simulink model "simulation"  (R2016b)
settings: Solver=FixedStepAuto  StartTime=0.0  StopTime=15  FixedStep=0.05  RelTol=1e-3
values from neighbouring files (symbols this model uses):
  AccReqTable = [ ... (first row only)    [paras_table.m]
  CC_Delta_V_Pos = [0    0.5   1   2   5   10   20   30]    [paras_table.m]
  CC_P_Arr_Pos = [0.6  0.6  0.5 0.4 0.2  0.15 0.1 0.08]    [paras_table.m]
  Delta_Acc = [ 0   0.5  0.8  1.2  1.6 2.0 3.0 5.0]    [paras_table.m]
  DeltaSArr = [-40 -35 -30 -25 -20 -18 -16 -14 -12 -10 -8 -6 -4 -2 0 2 4 6 8 10 12 14 16 18 20 25 30 35 40 45 50 60 70 80 90]    [paras_table.m]
  DeltaVArr = [-30 -28 -26 -24 -22 -20 -18 -16 -14 -12 -10  -9  -8  -7  -6  -5 -4 -3 -2 -1 0 1 2 3 4  5  6  7  8 9  10 12 14 16 18 20 22 24 26 28 30]    [paras_table.m]
  Ego_Acc_arr = [2    2     2   1.5    1]    [paras_table.m]
  Ego_dece_arr = [-5  -5     -4   -3.5 -2.5]    [paras_table.m]
  Ego_V_arr = [0    5     10   20    30]    [paras_table.m]
  Neg_Jerk = [-4   -4  -2.5 -2  -1]    [paras_table.m]
  Pos_Jerk = [0.5  0.8  1.2  1.8  2.0 2.5 3.0 3.0]    [paras_table.m]
  TTC_Arr = [0    10   20  40 100]    [paras_table.m]
settings Model: Creator=Administrator  LastModifiedBy=Administrator

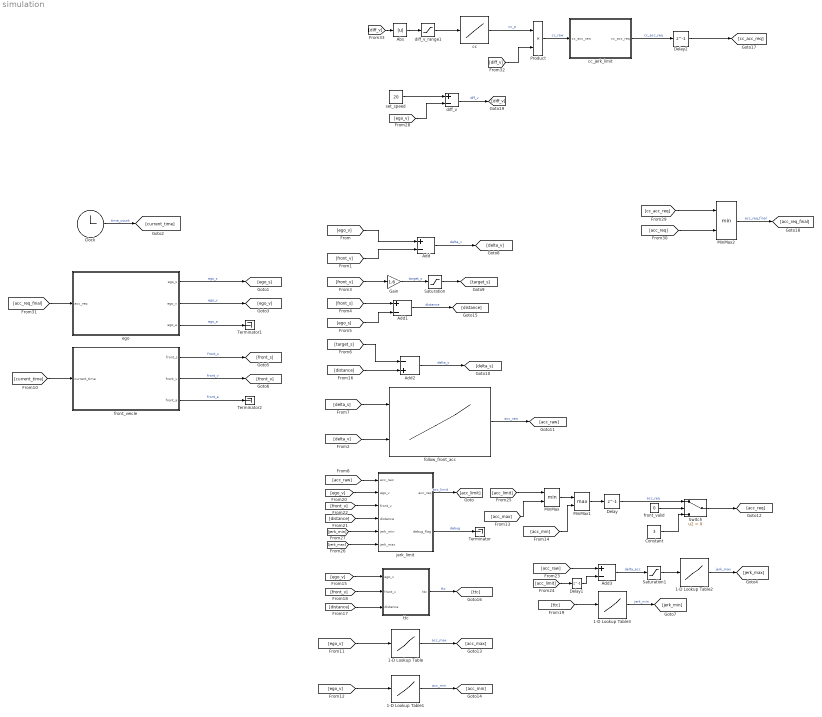
== system simulation ==
  1-D Lookup Table : Lookup_n-D  NumberOfTableDimensions=1  BreakpointsForDimension1=Ego_V_arr  Table=Ego_Acc_arr  InternalRulePriority=Speed  RndMeth=Simplest  InputSameDT=on
  1-D Lookup Table1 : Lookup_n-D  NumberOfTableDimensions=1  BreakpointsForDimension1=Ego_V_arr  Table=Ego_dece_arr  InternalRulePriority=Speed  RndMeth=Simplest  InputSameDT=on
  1-D Lookup Table2 : Lookup_n-D  NumberOfTableDimensions=1  BreakpointsForDimension1=Delta_Acc  Table=Pos_Jerk  InternalRulePriority=Speed  RndMeth=Simplest  InputSameDT=on
  1-D Lookup Table3 : Lookup_n-D  NumberOfTableDimensions=1  BreakpointsForDimension1=TTC_Arr  Table=Neg_Jerk  InternalRulePriority=Speed  RndMeth=Simplest  InputSameDT=on
  Abs : Abs
  Add : Sum  Inputs=+-
  Add1 : Sum  Inputs=+-
  Add2 : Sum  Inputs=-+
  Add3 : Sum  Inputs=+-
  Clock : Clock
  Constant : Constant  Value=3
  Delay : Delay  DelayLength=1  InitialCondition=0
  Delay1 : Delay  DelayLength=1  InitialCondition=0
  Delay2 : Delay  DelayLength=1  InitialCondition=0
  Gain : Gain  Gain=1.6
  MinMax : MinMax  Inputs=2
  MinMax1 : MinMax  Function=max  Inputs=2
  MinMax2 : MinMax  Inputs=2
  Product : Product
  Saturation : Saturate  UpperLimit=150  LowerLimit=3
  Saturation1 : Saturate  UpperLimit=5  LowerLimit=0
  Switch : Switch  Criteria=u2 > Threshold
  Terminator : Terminator
  Terminator1 : Terminator
  Terminator2 : Terminator
  cc : Lookup_n-D  NumberOfTableDimensions=1  BreakpointsForDimension1=CC_Delta_V_Pos  IndexSearchMethod=Linear search  Table=CC_P_Arr_Pos  InternalRulePriority=Speed  RndMeth=Simplest  InputSameDT=on
  cc_jerk_limit : MATLAB Function  TreatAsAtomicUnit=on
  diff_v : Sum  Inputs=+-
  diff_v_range1 : Saturate  UpperLimit=30  LowerLimit=0
  ego : MATLAB Function  TreatAsAtomicUnit=on
  "follow_front_acc " : Lookup_n-D  BreakpointsForDimension1=DeltaSArr  BreakpointsForDimension2=DeltaVArr  Table=AccReqTable  InternalRulePriority=Speed  RndMeth=Simplest  InputSameDT=on
  front_valid : Constant  Value=0
  front_veicle : MATLAB Function  TreatAsAtomicUnit=on
  jerk_limit : MATLAB Function  TreatAsAtomicUnit=on
  set_speed : Constant  Value=20
  ttc : MATLAB Function  TreatAsAtomicUnit=on
  wires:
  Clock/1 -> [current_time]  "time_count"
  ego/1(ego_s) -> [ego_s]  "ego_s"
  ego/2(ego_v) -> [ego_v]  "ego_v"
  ego/3(ego_a) -> Terminator1/1  "ego_a"
  front_veicle/1(front_s) -> [front_s]  "front_s"
  front_veicle/2(front_v) -> [front_v]  "front_v"
  front_veicle/3(front_a) -> Terminator2/1  "front_a"
  [ego_v] -> Add/1
  [front_v] -> Add/2
  Add/1 -> [delta_v]  "delta_v"
  [delta_v] -> "follow_front_acc "/2
  [front_v] -> Gain/1
  Gain/1 -> Saturation/1  "target_s"
  [front_s] -> Add1/1
  [ego_s] -> Add1/2
  [target_s] -> Add2/1
  Add2/1 -> [delta_s]  "delta_s"
  [delta_s] -> "follow_front_acc "/1
  "follow_front_acc "/1 -> [acc_raw]  "acc_raw"
  [acc_raw] -> jerk_limit/1(acc_raw)
  [acc_req_final] -> ego/1(acc_req)
  [current_time] -> front_veicle/1(current_time)
  [ego_v] -> 1-D Lookup Table/1
  1-D Lookup Table/1 -> [acc_max]  "acc_max"
  [ego_v] -> 1-D Lookup Table1/1
  1-D Lookup Table1/1 -> [acc_min]  "acc_min"
  [acc_max] -> MinMax/2
  MinMax/1 -> MinMax1/1
  [acc_min] -> MinMax1/2
  MinMax1/1 -> Delay/1
  Saturation/1 -> [target_s]
  [ego_v] -> ttc/1(ego_v)
  Add1/1 -> [distance]  "distance"
  [distance] -> Add2/2
  [distance] -> ttc/3(distance)
  [front_v] -> ttc/2(front_v)
  ttc/1(ttc) -> [ttc]  "ttc"
  [ttc] -> 1-D Lookup Table3/1
  [ego_v] -> jerk_limit/2(ego_v)
  [front_v] -> jerk_limit/3(front_v)
  [distance] -> jerk_limit/4(distance)
  jerk_limit/2(debug_flag) -> Terminator/1  "debug"
  [acc_raw] -> Add3/1
  jerk_limit/1(acc_req) -> [acc_limit]  "acc_limit"
  [acc_limit] -> MinMax/1
  Add3/1 -> Saturation1/1  "delta_acc"
  Saturation1/1 -> 1-D Lookup Table2/1
  1-D Lookup Table2/1 -> [jerk_max]  "jerk_max"
  [jerk_max] -> jerk_limit/6(jerk_max)
  1-D Lookup Table3/1 -> [jerk_min]  "jerk_min"
  [jerk_min] -> jerk_limit/5(jerk_min)
  [acc_limit] -> Delay1/1
  Delay1/1 -> Add3/2
  set_speed/1 -> diff_v/1
  [ego_v] -> diff_v/2
  cc/1 -> Product/1  "cc_p"
  cc_jerk_limit/1(cc_acc_req) -> Delay2/1  "cc_acc_req"
  [cc_acc_req] -> MinMax2/1
  [acc_req] -> MinMax2/2
  MinMax2/1 -> [acc_req_final]  "acc_req_final"
  front_valid/1 -> Switch/2
  Delay/1 -> Switch/1  "acc_req"
  Switch/1 -> [acc_req]
  Constant/1 -> Switch/3
  diff_v/1 -> [diff_v]  "dff_v"
  [diff_v] -> Product/2
  Product/1 -> cc_jerk_limit/1(cc_acc_raw)  "cc_raw"
  diff_v_range1/1 -> cc/1
  [diff_v] -> Abs/1
  Delay2/1 -> [cc_acc_req]
  Abs/1 -> diff_v_range1/1

== matlab function simulation/front_veicle ==
  data: current_time input; front_s output; front_v output; front_a output
function [front_s, front_v, front_a]= fcn(current_time)
persistent pre_front_s
persistent pre_front_v
persistent pre_front_a
%自车初始化
if isempty(pre_front_s)
    pre_front_s = 100;
end
if isempty(pre_front_v)
    pre_front_v = 0;
end
if isempty(pre_front_a)
    pre_front_a = 0;
end
dt = 0.05;
%% 前车匀速模型
front_a = pre_front_a;
front_v = pre_front_v + front_a * dt;
front_s = pre_front_s + pre_front_v * dt + 0.5 * front_a * dt^2;  


pre_front_s = front_s;
pre_front_v = front_v;
pre_front_a = front_a;
end

== matlab function simulation/ego ==
  data: acc_req input; ego_s output; ego_v output; ego_a output
function [ego_s, ego_v, ego_a]= fcn(acc_req)
persistent pre_ego_s
persistent pre_ego_v
persistent pre_ego_a
%自车初始化
if isempty(pre_ego_s)
    pre_ego_s = 0;
end
if isempty(pre_ego_v)
    pre_ego_v = 10;
end
if isempty(pre_ego_a)
    pre_ego_a = 0;
end
dt = 0.05;
%加速度响应
ego_a = pre_ego_a * 0.9 + acc_req * 0.1;
ego_v = pre_ego_v + ego_a * dt;
if ego_v < 0
    ego_v = 0;
end
ego_s = pre_ego_s + pre_ego_v * dt + 0.5 * ego_a * dt^2;  


pre_ego_s = ego_s;
pre_ego_v = ego_v;
pre_ego_a = ego_a;
end

== matlab function simulation/jerk_limit ==
  data: acc_raw input; acc_req output; ego_v input; front_v input; distance input; debug_flag output; jerk_min input; jerk_max input
function [acc_req, debug_flag] = fcn(acc_raw, ego_v, front_v, distance, jerk_min, jerk_max)
persistent pre_acc_req
if isempty(pre_acc_req)
    pre_acc_req = 0;
end
debug_flag = 0;
dt = 0.05;
neg_jerk = jerk_min;
if ((front_v - ego_v) > 3) && (distance < 1.0 * ego_v)
    if distance < 0.5 * ego_v
        neg_jerk = -4;
    elseif distance < 0.8 * ego_v
        neg_jerk = -3;
    else
        neg_jerk = -2;
    end
end
%正jerk
pos_jerk = jerk_max;
if acc_raw > pre_acc_req + pos_jerk * dt
    acc_req = pre_acc_req + pos_jerk * dt;
    debug_flag = debug_flag + 1;
elseif acc_raw < pre_acc_req + neg_jerk * dt
    acc_req = pre_acc_req + neg_jerk * dt;
    debug_flag = debug_flag + 2;
else
    acc_req = acc_raw;
    debug_flag = debug_flag + 4;
end
pre_acc_req = acc_req;
end

== matlab function simulation/ttc ==
  data: ego_v input; ttc output; front_v input; distance input
function ttc = fcn(ego_v, front_v, distance)
ttc = 100;
if (ego_v > front_v && distance > 0)
ttc = distance/(ego_v - front_v);
ttc = min(ttc, 100);
end

== matlab function simulation/cc_jerk_limit ==
  data: cc_acc_raw input; cc_acc_req output
function cc_acc_req = fcn(cc_acc_raw)
persistent pre_acc_req
if isempty(pre_acc_req)
    pre_acc_req = 0;
end
dt = 0.05;
pos_jerk = 1.0;
neg_jerk = -1.2;
if cc_acc_raw > pre_acc_req + pos_jerk * dt
    cc_acc_req = pre_acc_req + pos_jerk * dt;
elseif cc_acc_raw < pre_acc_req + neg_jerk * dt
    cc_acc_req = pre_acc_req + neg_jerk * dt;
else
    cc_acc_req = cc_acc_raw;
end
pre_acc_req = cc_acc_req;
end
